simulink model "LQR"  (Simulink 5.0)
settings: Solver=ode1  SolverMode=SingleTasking  StartTime=0.0  StopTime=inf  FixedStep=0.005  RelTol=1e-3
libraries: simulink x2
settings Model: LastModifiedBy=Administrator  ExtModeMexFile=rtwinext  ExtModeTrigDuration=100000  SimulationMode=external  LimitDataPoints=off  MaxDataPoints=20000  RTWSystemTargetFile=rtwin.tlc  RTWTemplateMakefile=rtwintmf  RTWOptions="-aCCOptimize=1 -aEnforceIntegerDowncast=1 -aExtMode=1 -aFoldNonRolledExpr=1 -aForceParamTrailComments=0 -aGenerateComments=1 -aGenerateReport=0 -aIncDataTypeInIds=0 -aIncHierarchyInIds=0 -aInlineInvariantSignals=0 -aInlineParameters=0 -aInlinedPrmAccess=\"Literals\" -aLocalBlockOutputs=1 -aMaxRTWIdLen=31 -aPrefixModelToSubsysFcnNames=1 -aRTWVerbose=1 -aRebuildAll=0 -aRollThreshold=5 -aShowEliminatedStatements=0"

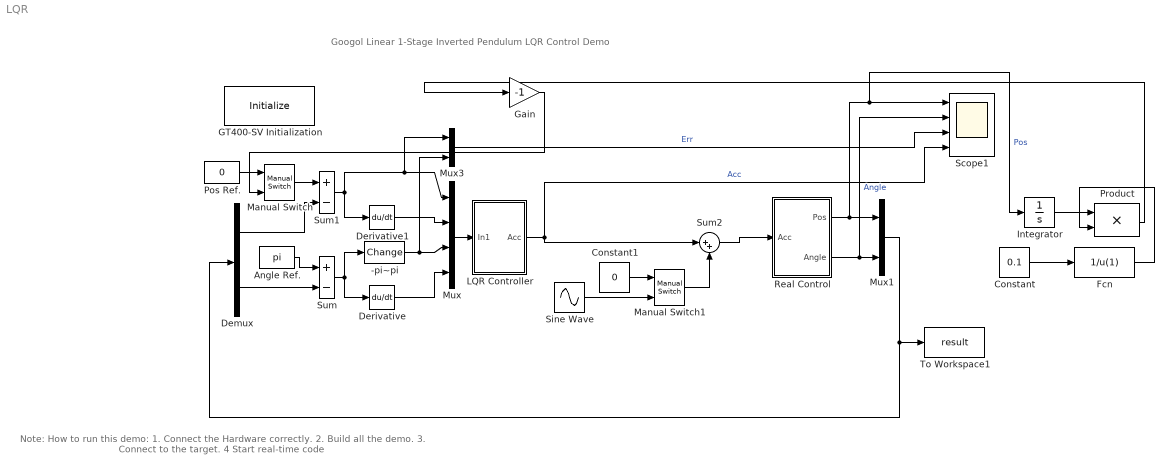
== system LQR ==
  note: Googol Linear 1-Stage Inverted Pendulum LQR Control Demo
  note: Note:
      |          How to run this demo:
      |          1.  Connect the Hardware correctly.
      |          2.  Build all the demo.
      |          3.  Connect to the target.
      |          4  Start real-time code
  " -pi~pi" : S-Function  FunctionName=Change
      mask Type: Change
      mask Description:
      | Change input signal between -pi and pi in 2*pi period.
      | Block input:
      |     any double.
      | Block output:
      |     between -pi and pi.
      | eg:
      |     If input is 1.5*pi, then output is -0.5*pi.
      mask Help:
      | This block, "change", input signal between -pi and pi in 2*pi period.
      | Block input:
      |     any double.
      | Block output:
      |     between -pi and pi.
      | eg:
      |     input is 1.5*pi, then output is -0.5*pi.
      mask Display: plot([0:0.01:2*pi],sin([0:0.01:2*pi]));
  Angle Ref. : Constant  Value=pi
  Constant : Constant  Value=0.1
  Constant1 : Constant  Value=0
  Demux : Demux  Outputs=2
  Derivative : Derivative
  Derivative1 : Derivative
  Fcn : Fcn  Expr=1/u(1)
  GT400-SV Initialization : S-Function  Priority=0  FunctionName=Initialize  Parameters=openloop  mask(Initialize){openloop=0}
      mask prompts: openloop "Control loop:"
      mask help:
      | Initializing the googol GT400-SV motion control board.
      | Block parameter:
      |     Control loop:
      |          0: closed-loop control.
      |          1: opened-loop control.
      mask Help: This initialize block initializes the googol GT400-SV motion control board.
      mask Display: disp('Initialize \nGT400-SV');
  Gain : Gain  Gain=-1  SaturateOnIntegerOverflow=on
  Integrator : Integrator
  LQR Controller : Subsystem  mask{x=-36.51, xdot=-23.62, angle=87.97, angledot=16.08}
      mask prompts: x "Kx"; xdot "Kx'"; angle "Ka"; angledot "Ka'"
  Manual Switch : simulink/Signal Routing/Manual Switch  sw=0  action=0
  Manual Switch1 : simulink/Signal Routing/Manual Switch  sw=1  action=0
  Mux : Mux
  Mux1 : Mux  Inputs=2
  Mux3 : Mux  Inputs=2
  Pos Ref. : Constant  Value=0
  Product : Product  SaturateOnIntegerOverflow=on
  Real Control : Subsystem
  Scope1 : Scope  NumInputPorts=4
      settings: TickLabels=on  TimeRange=100  YMin=-0.2~0~-1~-100  YMax=0.3~4~4~300  SaveName=PosData  MaxDataPoints=20000
  Sine Wave : Sin  SampleTime=0
  Sum : Sum  Inputs=+-  SaturateOnIntegerOverflow=on
  Sum1 : Sum  Inputs=+-  SaturateOnIntegerOverflow=on
  Sum2 : Sum  Inputs=|++  SaturateOnIntegerOverflow=on
  To Workspace1 : ToWorkspace  VariableName=result  SampleTime=0.005  SaveFormat=Array
  wires:
  Mux/1 -> LQR Controller/1(In1)
  Mux1/1 -> To Workspace1/1, Demux/1
  Sum/1 -> Derivative/1, " -pi~pi"/1
  Demux/2 -> Sum/2
  Demux/1 -> Sum1/2
  Sum1/1 -> Derivative1/1, Mux/1, Mux3/1
  Real Control/2(Angle) -> Mux1/2, Scope1/2  "Angle"
  Angle Ref./1 -> Sum/1
  " -pi~pi"/1 -> Mux/3, Mux3/2
  Real Control/1(Pos) -> Mux1/1, Scope1/1, Integrator/1  "Pos"
  Derivative/1 -> Mux/4
  Derivative1/1 -> Mux/2
  LQR Controller/1(Acc) -> Scope1/4, Sum2/1  "Acc"
  Mux3/1 -> Scope1/3  "Err"
  Manual Switch/1 -> Sum1/1
  Pos Ref./1 -> Manual Switch/1
  Gain/1 -> Manual Switch/2
  Manual Switch1/1 -> Sum2/2
  Sum2/1 -> Real Control/1(Acc)
  Constant1/1 -> Manual Switch1/1
  Sine Wave/1 -> Manual Switch1/2
  Constant/1 -> Fcn/1
  Integrator/1 -> Product/1
  Fcn/1 -> Product/2
  Product/1 -> Gain/1

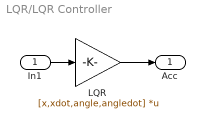
== system LQR/LQR Controller ==
  In1 : Inport
  LQR : Gain  Gain=[x,xdot,angle,angledot]  Multiplication=Matrix(K*u)  SaturateOnIntegerOverflow=on
  Acc : Outport
  wires:
  LQR/1 -> Acc/1
  In1/1 -> LQR/1

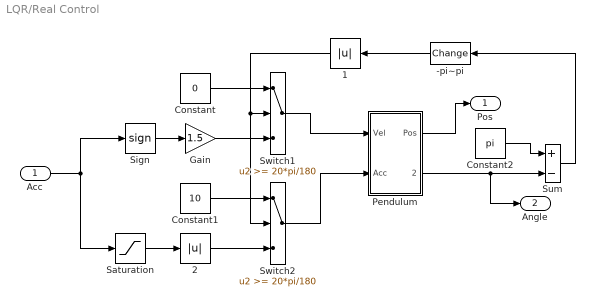
== system LQR/Real Control ==
  Acc : Inport
  " -pi~pi" : S-Function  Orientation=left  AncestorBlock=googolbox/GT-400-SV Block Library/ -pi~pi  FunctionName=Change
      mask Type: Change
      mask Description:
      | Change input signal between -pi and pi in 2*pi period.
      | Block input:
      |     any double.
      | Block output:
      |     between -pi and pi.
      | eg:
      |     If input is 1.5*pi, then output is -0.5*pi.
      mask Help:
      | This block, "change", input signal between -pi and pi in 2*pi period.
      | Block input:
      |     any double.
      | Block output:
      |     between -pi and pi.
      | eg:
      |     input is 1.5*pi, then output is -0.5*pi.
      mask Display: plot([0:0.01:2*pi],sin([0:0.01:2*pi]));
  " 1" : Abs  Orientation=left  SaturateOnIntegerOverflow=on
  " 2" : Abs  SaturateOnIntegerOverflow=on
  Constant : Constant  Value=0
  Constant1 : Constant  Value=10
  Constant2 : Constant  Value=pi
  Gain : Gain  Gain=1.5  SaturateOnIntegerOverflow=on
  Pendulum : Subsystem
  Saturation : Saturate  UpperLimit=15  LowerLimit=-15
  Sign : Signum
  Sum : Sum  Inputs=+-  SaturateOnIntegerOverflow=on
  Switch1 : Switch  Threshold=20*pi/180  SaturateOnIntegerOverflow=on
  Switch2 : Switch  Threshold=20*pi/180  SaturateOnIntegerOverflow=on
  Pos : Outport
  Angle : Outport  Port=2
  wires:
  Acc/1 -> Saturation/1, Sign/1
  Sign/1 -> Gain/1
  Pendulum/2(Angle) -> Angle/1, Sum/2
  Pendulum/1(Pos) -> Pos/1
  Saturation/1 -> " 2"/1
  " 1"/1 -> Switch2/2, Switch1/2
  " -pi~pi"/1 -> " 1"/1
  Switch2/1 -> Pendulum/2(Acc)
  Switch1/1 -> Pendulum/1(Vel)
  Constant2/1 -> Sum/1
  Sum/1 -> " -pi~pi"/1
  Gain/1 -> Switch1/3
  Constant/1 -> Switch1/1
  " 2"/1 -> Switch2/3
  Constant1/1 -> Switch2/1

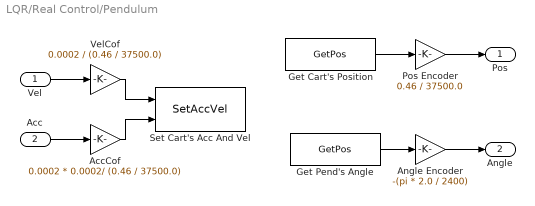
== system LQR/Real Control/Pendulum ==
  Vel : Inport
  Acc : Inport  Port=2
  AccCof : Gain  Gain=0.0002 * 0.0002/ (0.46 / 37500.0)  SaturateOnIntegerOverflow=on
  Angle Encoder : Gain  Gain=-(pi * 2.0 / 2400)  SaturateOnIntegerOverflow=on
  Get Cart's Position : S-Function  Priority=1  FunctionName=GetPos  Parameters=axis  mask(GetPos){axis=1}
      mask prompts: axis "Axis number:"
      mask help:
      | Getting the current axis position value in encoder' counts.
      | Block parameter:
      |     Axis number:  must be between 1 and 6, default is 1.
      | Block output:
      |     1~4: current axis' encoder reading counts.
      |     5/6: assistant encoder 1/2 reading counts.
      mask Help:
      | This block, GetPos, is intended for getting the current axis position value in encoder' counts. This value represents the actual position for the axis
      | at the current sample time. This command operates for all profile modes.
      | The value returned is a 32-bit signed number with units of counts.
      | The range is -1,073,741,824 to 1,073,741,823.
      | 
      | You can recalculate obtained value into meter units via multiplication by the scaler coefficient .
      | 
      | Block parameter:
      |     Axis number:  must be between 1 and 4, default is 1.
      | Block input: none.
      | Block output:
      |         1~4: current axis' encoder reading counts.
      |         5/6: assistant encoder 1/2 reading counts.
      mask Display:
      | disp('GetPos');
      | port_label('output', 1, 'Pos');
  Get Pend's Angle : S-Function  Priority=1  FunctionName=GetPos  Parameters=axis  mask(GetPos){axis=2}
      mask prompts: axis "Axis number:"
      mask help:
      | Getting the current axis position value in encoder' counts.
      | Block parameter:
      |     Axis number:  must be between 1 and 6, default is 1.
      | Block output:
      |     1~4: current axis' encoder reading counts.
      |     5/6: assistant encoder 1/2 reading counts.
      mask Help:
      | This block, GetPos, is intended for getting the current axis position value in encoder' counts. This value represents the actual position for the axis
      | at the current sample time. This command operates for all profile modes.
      | The value returned is a 32-bit signed number with units of counts.
      | The range is -1,073,741,824 to 1,073,741,823.
      | 
      | You can recalculate obtained value into meter units via multiplication by the scaler coefficient .
      | 
      | Block parameter:
      |     Axis number:  must be between 1 and 4, default is 1.
      | Block input: none.
      | Block output:
      |         1~4: current axis' encoder reading counts.
      |         5/6: assistant encoder 1/2 reading counts.
      mask Display:
      | disp('GetPos');
      | port_label('output', 1, 'Pos');
  Pos Encoder : Gain  Gain=0.46 / 37500.0  SaturateOnIntegerOverflow=on
  Set Cart's Acc And Vel : S-Function  Priority=1  FunctionName=SetAccVel  Parameters=axis, vel, pos  mask(SetAccVel){axis=1, vel=0.1, pos=250000}
      mask prompts: axis "Axis number:"; vel "Back velocity:"; pos "Back position:"
      mask help:
      | Setting the current axis' acceleration and velocity.
      |
      | Block parameter:
      |     Axis number:
      |         must be between 1 and 4, default is 1;
      |     Back velocity:
      |          After the current axis' limit reached, the moter will moves back as this  velocity, it must >=0;
      |     Back position:
      |          After the current axis' limit reached, the moter will moves back to this postion relative to limit, it must >=0;
      |
      | Block input:
      |     Vel: the current axis' velocity.
      |     Acc: the current axis' acceleration.
      mask Help:
      | This SetAccVel bolck Sets the current axis' acceleration and velocity.
      | Block parameter:
      |     Axis number: must be between 1 and 4, default is 1.
      | Block input:
      |     Vel: the current axis' velocity.
      |     Acc: the current axis' acceleration.
      mask Display:
      | disp('          SetAccVel');
      | port_label('input', 1, 'Vel');
      | port_label('input', 2, 'Acc');
  VelCof : Gain  Gain=0.0002 / (0.46 / 37500.0)  SaturateOnIntegerOverflow=on
  Pos : Outport
  Angle : Outport  Port=2
  wires:
  Get Cart's Position/1 -> Pos Encoder/1
  Vel/1 -> VelCof/1
  Acc/1 -> AccCof/1
  Get Pend's Angle/1 -> Angle Encoder/1
  Pos Encoder/1 -> Pos/1
  Angle Encoder/1 -> Angle/1
  VelCof/1 -> Set Cart's Acc And Vel/1
  AccCof/1 -> Set Cart's Acc And Vel/2
